simulink model "lab3es1ver2"  (R2022a)
settings: Solver=VariableStepAuto  StartTime=0.0  StopTime=10.0  RelTol=1e-3
settings Model: Creator=bonvoltnuovo  LastModifiedBy=bonaventur
settings DebuggingCC: UnconnectedInputMsg=warning  UnconnectedOutputMsg=warning  UnconnectedLineMsg=warning
settings RTWCC: DLArmComputeVersion=19.05

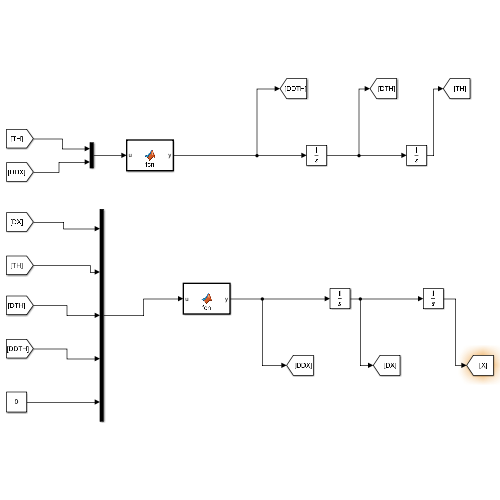
[thumbnail: Simulink's stored preview of the top-level diagram]
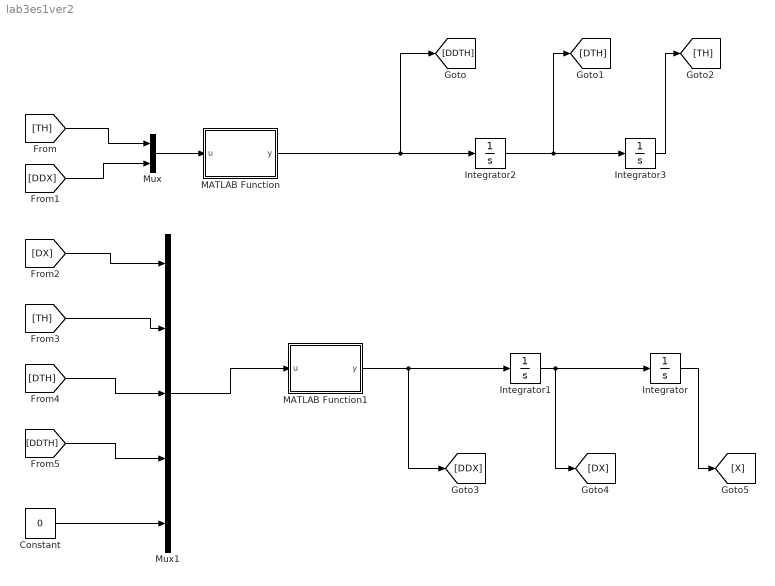
== system lab3es1ver2 ==
  Constant : Constant  Value=0
  Integrator{,1..3} (4 alike) : Integrator
  MATLAB Function : MATLAB Function  TreatAsAtomicUnit=on
  MATLAB Function1 : MATLAB Function  TreatAsAtomicUnit=on
  Mux : Mux  Inputs=2
  Mux1 : Mux  Inputs=5
  wires:
  [DDX] -> Mux/2
  Mux/1 -> MATLAB Function/1(u)
  [TH] -> Mux/1
  Integrator2/1 -> Integrator3/1, [DTH]
  Integrator3/1 -> [TH]
  MATLAB Function/1(y) -> [DDTH], Integrator2/1
  Constant/1 -> Mux1/5
  [DTH] -> Mux1/3
  [DX] -> Mux1/1
  [DDTH] -> Mux1/4
  Integrator1/1 -> Integrator/1, [DX]
  Integrator/1 -> [X]
  [TH] -> Mux1/2
  Mux1/1 -> MATLAB Function1/1(u)
  MATLAB Function1/1(y) -> [DDX], Integrator1/1

== matlab function lab3es1ver2/MATLAB Function ==
  data: u input; y output
function y = fcn(u)
M=0.455; %[kg] Cart mass
m=0.21; %[kg] Pendulum mass
l=0.305; %[m] Pendulum half-length 
I=1/3*m*l^2; %[kg*m^2]Pendulum moment of inertia 
b=1.0; %[N*s/m] Cart viscous friction coefficient
g=9.81;
Ie=I+m*l^2;
y = (m*l*cos(u(1))*u(2)+m*g*l*sin(u(1)))/Ie;
end

== matlab function lab3es1ver2/MATLAB Function1 ==
  data: u input; y output
function y = fcn(u)

y = u(1);
end
